simulink model "flujos_simulacion"  (Simulink 7.5)
settings: Solver=ode45  StartTime=0.0  StopTime=1000  RelTol=1e-3
InitFcn:
  | 'para_inv_prechancado';
  | 'mmmmmm';
values from neighbouring files (symbols this model uses):
  D = 0.8    [D.mat]    (also in Flujos_verificacion2.m; Flujos_verificacion3.m; Fujos_verificacion.m)
  Gs6 = 26.683353    [Flujos_verificacion2.m]    (also in Flujos_verificacion3.m; Fujos_verificacion.m)
  L = 0.25    [Flujos_verificacion2.m]    (also in Flujos_verificacion3.m; Fujos_verificacion.m; L.mat)
  s0 = 0.019    [Flujos_verificacion2.m]    (also in Flujos_verificacion3.m; Fujos_verificacion.m)
undefined symbols (not defined in the file or in its folder): roa, U, vol3, vol4, vol5
settings Model: Creator=Fer  LastModifiedBy=Fer

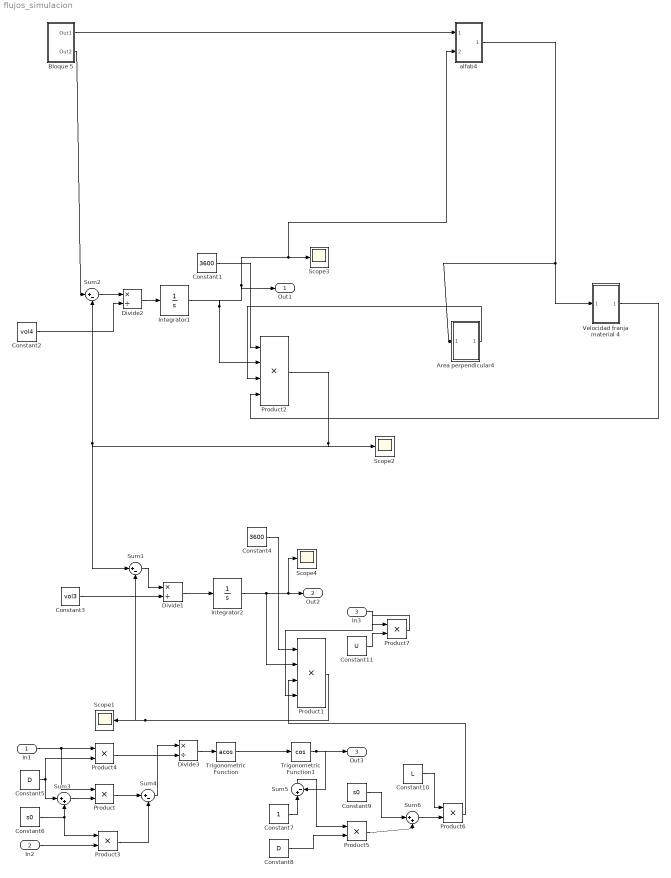
== system flujos_simulacion ==
  In1 : Inport  OutDataType=fixdt(1, 16)  OutScaling=2^0
  In2 : Inport  Port=2  OutDataType=fixdt(1, 16)  OutScaling=2^0
  In3 : Inport  Port=3  OutDataType=fixdt(1, 16)  OutScaling=2^0
  Area perpendicular4 : Subsystem
  Bloque 5 : Subsystem
  Constant1 : Constant  Value=3600  OutDataType=fixdt(1, 16)  OutScaling=2^0
  Constant10 : Constant  Value=L  OutDataType=fixdt(1, 16)  OutScaling=2^0
  Constant11 : Constant  Value=U  OutDataType=fixdt(1, 16)  OutScaling=2^0
  Constant2 : Constant  Value=vol4  OutDataType=fixdt(1, 16)  OutScaling=2^0
  Constant3 : Constant  Value=vol3  OutDataType=fixdt(1, 16)  OutScaling=2^0
  Constant4 : Constant  Value=3600  OutDataType=fixdt(1, 16)  OutScaling=2^0
  Constant5 : Constant  Value=D  OutDataType=fixdt(1, 16)  OutScaling=2^0
  Constant6 : Constant  Value=s0  OutDataType=fixdt(1, 16)  OutScaling=2^0
  Constant7 : Constant  OutDataType=fixdt(1, 16)  OutScaling=2^0
  Constant8 : Constant  Value=D  OutDataType=fixdt(1, 16)  OutScaling=2^0
  Constant9 : Constant  Value=s0  OutDataType=fixdt(1, 16)  OutScaling=2^0
  Divide1 : Product  Inputs=*/  OutDataType=fixdt(1, 16)  OutScaling=2^-10
  Divide2 : Product  Inputs=*/  OutDataType=fixdt(1, 16)  OutScaling=2^-10
  Divide3 : Product  Inputs=*/  OutDataType=fixdt(1, 16)  OutScaling=2^-10
  Integrator1 : Integrator  InitialCondition=2.1
  Integrator2 : Integrator  InitialCondition=2.1
  Product{,3..7} (6 alike) : Product  OutDataType=fixdt(1, 16)  OutScaling=2^0  RndMeth=Zero
  Product1 : Product  Inputs=4  OutDataType=fixdt(1, 16)  OutScaling=2^0  RndMeth=Zero
  Product2 : Product  Inputs=4  OutDataType=fixdt(1, 16)  OutScaling=2^0  RndMeth=Zero
  Scope{1..4} (4 alike) : Scope
      Scope1 settings: SaveName=ScopeData4
      Scope2 settings: SaveName=ScopeData2
      Scope3 settings: SaveName=ScopeData3
      Scope4 settings: SaveName=ScopeData5
  Sum{1..2,4..5} (4 alike) : Sum  Inputs=|+-  OutDataType=fixdt(1, 16)  OutScaling=2^0
  Sum3 : Sum  Inputs=|++  OutDataType=fixdt(1, 16)  OutScaling=2^0
  Sum6 : Sum  Inputs=|++  OutDataType=fixdt(1, 16)  OutScaling=2^0
  Trigonometric Function : Trigonometry  Operator=acos
  Trigonometric Function1 : Trigonometry  Operator=cos
  Velocidad franja material 4 : Subsystem
  alfab4 : Subsystem
  Out1 : Outport  OutDataType=fixdt(1, 16)  OutScaling=2^0
  Out2 : Outport  Port=2  OutDataType=fixdt(1, 16)  OutScaling=2^0
  Out3 : Outport  Port=3  OutDataType=fixdt(1, 16)  OutScaling=2^0
  wires:
  Sum2/1 -> Divide2/1
  Constant2/1 -> Divide2/2
  Divide2/1 -> Integrator1/1
  Constant1/1 -> Product2/1
  Integrator1/1 -> Product2/2, Scope3/1, alfab4/2(In2), Out1/1
  alfab4/1(Out1) -> Area perpendicular4/1(In1), Velocidad franja material 4/1(In1)
  Area perpendicular4/1(Out1) -> Product2/3
  Velocidad franja material 4/1(Out1) -> Product2/4
  Bloque 5/1(Out1) -> alfab4/1(In1)
  Bloque 5/2(Out2) -> Sum2/1
  Product2/1 -> Scope2/1, Sum2/2, Sum1/1
  Constant3/1 -> Divide1/2
  Divide1/1 -> Integrator2/1
  Integrator2/1 -> Product1/2, Out2/1, Scope4/1
  Constant4/1 -> Product1/1
  Product1/1 -> Sum1/2, Scope1/1
  Sum1/1 -> Divide1/1
  Constant5/1 -> Sum3/1, Product4/2
  Constant6/1 -> Sum3/2, Product3/1
  Sum3/1 -> Product/2
  In1/1 -> Product/1, Product4/1
  In2/1 -> Product3/2
  Product/1 -> Sum4/1
  Product3/1 -> Sum4/2
  Sum4/1 -> Divide3/1
  Product4/1 -> Divide3/2
  Divide3/1 -> Trigonometric Function/1
  Constant7/1 -> Sum5/1
  Trigonometric Function/1 -> Trigonometric Function1/1
  Trigonometric Function1/1 -> Sum5/2, Out3/1
  Constant8/1 -> Product5/2
  Sum5/1 -> Product5/1
  Constant9/1 -> Sum6/1
  Product5/1 -> Sum6/2
  Constant10/1 -> Product6/1
  Sum6/1 -> Product6/2
  Product6/1 -> Product1/3
  In3/1 -> Product7/1
  Constant11/1 -> Product7/2
  Product7/1 -> Product1/4

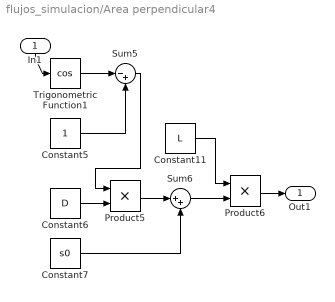
== system flujos_simulacion/Area perpendicular4 ==
  In1 : Inport
  Constant11 : Constant  Value=L  OutDataType=fixdt(1, 16)  OutScaling=2^0
  Constant5 : Constant  OutDataType=fixdt(1, 16)  OutScaling=2^0
  Constant6 : Constant  Value=D  OutDataType=fixdt(1, 16)  OutScaling=2^0
  Constant7 : Constant  Value=s0  OutDataType=fixdt(1, 16)  OutScaling=2^0
  Product5 : Product  OutDataType=fixdt(1, 16)  OutScaling=2^0  RndMeth=Zero
  Product6 : Product  OutDataType=fixdt(1, 16)  OutScaling=2^0  RndMeth=Zero
  Sum5 : Sum  Inputs=|-+  OutDataType=fixdt(1, 16)  OutScaling=2^0
  Sum6 : Sum  Inputs=|++  OutDataType=fixdt(1, 16)  OutScaling=2^0
  Trigonometric Function1 : Trigonometry  Operator=cos
  Out1 : Outport
  wires:
  Trigonometric Function1/1 -> Sum5/1
  Constant5/1 -> Sum5/2
  Constant6/1 -> Product5/2
  Sum5/1 -> Product5/1
  Product5/1 -> Sum6/1
  Constant7/1 -> Sum6/2
  Sum6/1 -> Product6/2
  Constant11/1 -> Product6/1
  In1/1 -> Trigonometric Function1/1
  Product6/1 -> Out1/1

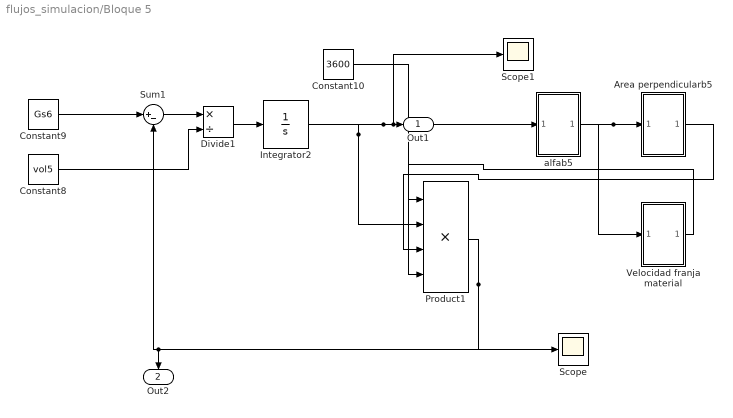
== system flujos_simulacion/Bloque 5 ==
  Area perpendicularb5 : Subsystem
  Constant10 : Constant  Value=3600  OutDataType=fixdt(1, 16)  OutScaling=2^0
  Constant8 : Constant  Value=vol5  OutDataType=fixdt(1, 16)  OutScaling=2^0
  Constant9 : Constant  Value=Gs6  OutDataType=fixdt(1, 16)  OutScaling=2^0
  Divide1 : Product  Inputs=*/  OutDataType=fixdt(1, 16)  OutScaling=2^-10
  Integrator2 : Integrator  InitialCondition=2.1
  Product1 : Product  Inputs=4  OutDataType=fixdt(1, 16)  OutScaling=2^0  RndMeth=Zero
  Scope : Scope
  Scope1 : Scope
  Sum1 : Sum  Inputs=|+-  OutDataType=fixdt(1, 16)  OutScaling=2^0
  Velocidad franja material : Subsystem
  alfab5 : Subsystem
  Out1 : Outport
  Out2 : Outport  Port=2
  wires:
  Constant9/1 -> Sum1/1
  Sum1/1 -> Divide1/1
  Constant8/1 -> Divide1/2
  Divide1/1 -> Integrator2/1
  Constant10/1 -> Product1/1
  Integrator2/1 -> Product1/2, alfab5/1(In1), Scope1/1, Out1/1
  Product1/1 -> Scope/1, Sum1/2, Out2/1
  alfab5/1(Out1) -> Area perpendicularb5/1(In1), Velocidad franja material/1(In1)
  Area perpendicularb5/1(Out1) -> Product1/3
  Velocidad franja material/1(Out1) -> Product1/4

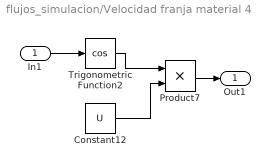
== system flujos_simulacion/Velocidad franja material 4 ==
  In1 : Inport
  Constant12 : Constant  Value=U  OutDataType=fixdt(1, 16)  OutScaling=2^0
  Product7 : Product  OutDataType=fixdt(1, 16)  OutScaling=2^0  RndMeth=Zero
  Trigonometric Function2 : Trigonometry  Operator=cos
  Out1 : Outport
  wires:
  Trigonometric Function2/1 -> Product7/1
  Constant12/1 -> Product7/2
  In1/1 -> Trigonometric Function2/1
  Product7/1 -> Out1/1

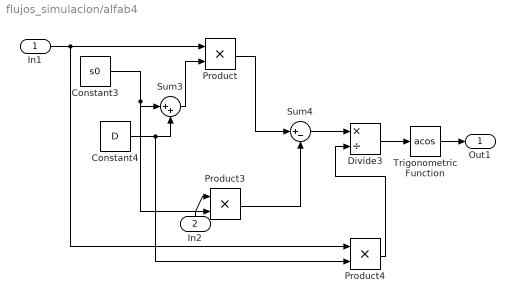
== system flujos_simulacion/alfab4 ==
  In1 : Inport
  In2 : Inport  Port=2
  Constant3 : Constant  Value=s0  OutDataType=fixdt(1, 16)  OutScaling=2^0
  Constant4 : Constant  Value=D  OutDataType=fixdt(1, 16)  OutScaling=2^0
  Divide3 : Product  Inputs=*/  OutDataType=fixdt(1, 16)  OutScaling=2^-10
  Product : Product  OutDataType=fixdt(1, 16)  OutScaling=2^0  RndMeth=Zero
  Product3 : Product  OutDataType=fixdt(1, 16)  OutScaling=2^0  RndMeth=Zero
  Product4 : Product  OutDataType=fixdt(1, 16)  OutScaling=2^0  RndMeth=Zero
  Sum3 : Sum  Inputs=|++  OutDataType=fixdt(1, 16)  OutScaling=2^0
  Sum4 : Sum  Inputs=|+-  OutDataType=fixdt(1, 16)  OutScaling=2^0
  Trigonometric Function : Trigonometry  Operator=acos
  Out1 : Outport
  wires:
  Constant3/1 -> Sum3/1, Product3/2
  Constant4/1 -> Sum3/2, Product4/2
  Sum3/1 -> Product/2
  Product/1 -> Sum4/1
  Product3/1 -> Sum4/2
  Sum4/1 -> Divide3/1
  Product4/1 -> Divide3/2
  Divide3/1 -> Trigonometric Function/1
  In1/1 -> Product/1, Product4/1
  In2/1 -> Product3/1
  Trigonometric Function/1 -> Out1/1

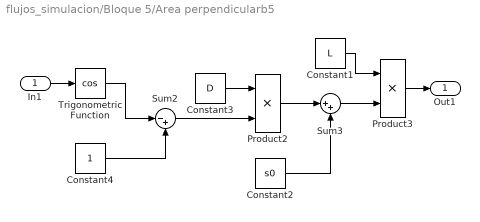
== system flujos_simulacion/Bloque 5/Area perpendicularb5 ==
  In1 : Inport
  Constant1 : Constant  Value=L  OutDataType=fixdt(1, 16)  OutScaling=2^0
  Constant2 : Constant  Value=s0  OutDataType=fixdt(1, 16)  OutScaling=2^0
  Constant3 : Constant  Value=D  OutDataType=fixdt(1, 16)  OutScaling=2^0
  Constant4 : Constant  OutDataType=fixdt(1, 16)  OutScaling=2^0
  Product2 : Product  OutDataType=fixdt(1, 16)  OutScaling=2^0  RndMeth=Zero
  Product3 : Product  OutDataType=fixdt(1, 16)  OutScaling=2^0  RndMeth=Zero
  Sum2 : Sum  Inputs=|-+  OutDataType=fixdt(1, 16)  OutScaling=2^0
  Sum3 : Sum  Inputs=|++  OutDataType=fixdt(1, 16)  OutScaling=2^0
  Trigonometric Function : Trigonometry  Operator=cos
  Out1 : Outport
  wires:
  Trigonometric Function/1 -> Sum2/1
  Constant4/1 -> Sum2/2
  Constant3/1 -> Product2/1
  Sum2/1 -> Product2/2
  Product2/1 -> Sum3/1
  Constant2/1 -> Sum3/2
  Constant1/1 -> Product3/1
  Sum3/1 -> Product3/2
  In1/1 -> Trigonometric Function/1
  Product3/1 -> Out1/1

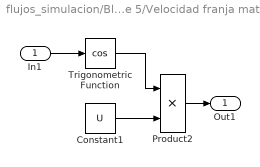
== system flujos_simulacion/Bloque 5/Velocidad franja material ==
  In1 : Inport
  Constant1 : Constant  Value=U  OutDataType=fixdt(1, 16)  OutScaling=2^0
  Product2 : Product  OutDataType=fixdt(1, 16)  OutScaling=2^0  RndMeth=Zero
  Trigonometric Function : Trigonometry  Operator=cos
  Out1 : Outport
  wires:
  Constant1/1 -> Product2/2
  Trigonometric Function/1 -> Product2/1
  In1/1 -> Trigonometric Function/1
  Product2/1 -> Out1/1

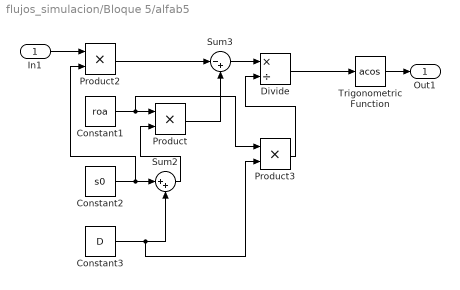
== system flujos_simulacion/Bloque 5/alfab5 ==
  In1 : Inport
  Constant1 : Constant  Value=roa  OutDataType=fixdt(1, 16)  OutScaling=2^0
  Constant2 : Constant  Value=s0  OutDataType=fixdt(1, 16)  OutScaling=2^0
  Constant3 : Constant  Value=D  OutDataType=fixdt(1, 16)  OutScaling=2^0
  Divide : Product  Inputs=*/  OutDataType=fixdt(1, 16)  OutScaling=2^-10
  Product : Product  OutDataType=fixdt(1, 16)  OutScaling=2^0  RndMeth=Zero
  Product2 : Product  OutDataType=fixdt(1, 16)  OutScaling=2^0  RndMeth=Zero
  Product3 : Product  OutDataType=fixdt(1, 16)  OutScaling=2^0  RndMeth=Zero
  Sum2 : Sum  Inputs=|++  OutDataType=fixdt(1, 16)  OutScaling=2^0
  Sum3 : Sum  Inputs=|-+  OutDataType=fixdt(1, 16)  OutScaling=2^0
  Trigonometric Function : Trigonometry  Operator=acos
  Out1 : Outport
  wires:
  Constant1/1 -> Product/1, Product3/1
  Constant2/1 -> Sum2/1, Product2/2
  Constant3/1 -> Sum2/2, Product3/2
  Sum2/1 -> Product/2
  Product2/1 -> Sum3/1
  Product/1 -> Sum3/2
  Sum3/1 -> Divide/1
  Product3/1 -> Divide/2
  Divide/1 -> Trigonometric Function/1
  In1/1 -> Product2/1
  Trigonometric Function/1 -> Out1/1
